simulink model "plane"  (R2023b)
settings: Solver=FixedStepDiscrete  StartTime=0.0  StopTime=17.0  FixedStep=1  RelTol=1e-3  EnableMultiTasking=on
libraries: simulink x3
settings Model: Creator=yueyue  LastModifiedBy=yueyue

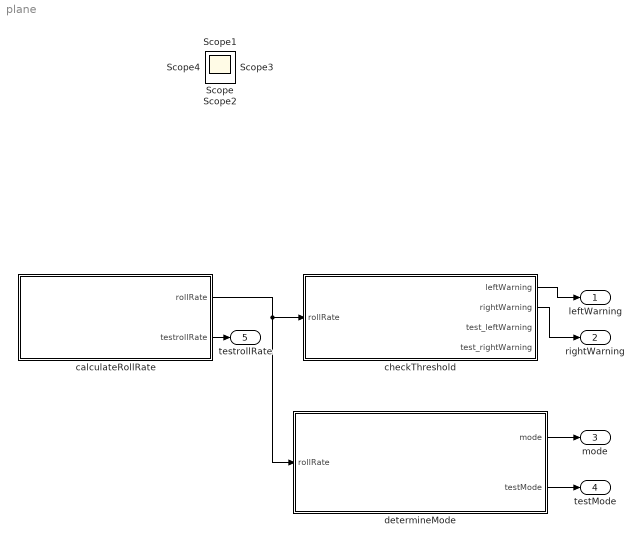
== system plane ==
  calculateRollRate : Subsystem
  checkThreshold : Subsystem
  determineMode : Subsystem
  leftWarning : Outport
  rightWarning : Outport  Port=2
  mode : Outport  Port=3
  testMode : Outport  Port=4
  testrollRate : Outport  Port=5
  Scope{,1..4} (5 alike) : Scope
  wires:
  calculateRollRate/1(rollRate) -> determineMode/1(rollRate), checkThreshold/1(rollRate)
  checkThreshold/1(leftWarning) -> leftWarning/1
  checkThreshold/2(rightWarning) -> rightWarning/1
  determineMode/1(mode) -> mode/1
  determineMode/2(testMode) -> testMode/1
  calculateRollRate/2(testrollRate) -> testrollRate/1

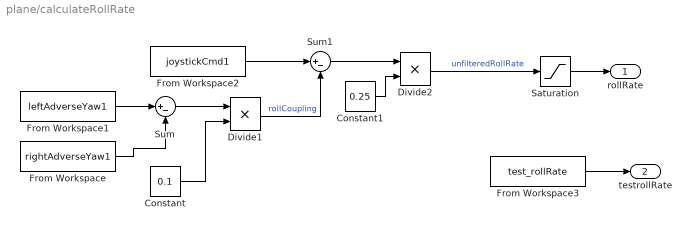
== system plane/calculateRollRate ==
  Constant : Constant  Value=0.1
  Constant1 : Constant  Value=0.25
  Divide1 : Product  Inputs=**
  Divide2 : Product  Inputs=**
  From Workspace : FromWorkspace  VariableName=rightAdverseYaw1  SampleTime=1
  From Workspace1 : FromWorkspace  VariableName=leftAdverseYaw1  SampleTime=1
  From Workspace2 : FromWorkspace  VariableName=joystickCmd1  SampleTime=1
  From Workspace3 : FromWorkspace  VariableName=test_rollRate  SampleTime=1
  Saturation : Saturate  UpperLimit=25.0  LowerLimit=-25.0  ZeroCross=off
  Sum : Sum  Inputs=|+-
  Sum1 : Sum  Inputs=|+-
  rollRate : Outport
  testrollRate : Outport  Port=2
  wires:
  Sum/1 -> Divide1/1
  Constant/1 -> Divide1/2
  Divide1/1 -> Sum1/2  "rollCoupling"
  Sum1/1 -> Divide2/1
  Constant1/1 -> Divide2/2
  Divide2/1 -> Saturation/1  "unfilteredRollRate"
  Saturation/1 -> rollRate/1
  From Workspace/1 -> Sum/2
  From Workspace1/1 -> Sum/1
  From Workspace2/1 -> Sum1/1
  From Workspace3/1 -> testrollRate/1

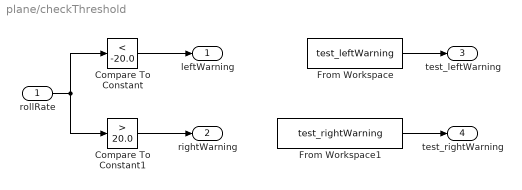
== system plane/checkThreshold ==
  rollRate : Inport
  Compare To Constant : simulink/Logic and Bit Operations/Compare To Constant  relop=<  const=-20.0  OutDataTypeStr=boolean
  Compare To Constant1 : simulink/Logic and Bit Operations/Compare To Constant  relop=>  const=20.0  OutDataTypeStr=boolean
  From Workspace : FromWorkspace  VariableName=test_leftWarning  SampleTime=1
  From Workspace1 : FromWorkspace  VariableName=test_rightWarning  SampleTime=1
  leftWarning : Outport
  rightWarning : Outport  Port=2
  test_leftWarning : Outport  Port=3
  test_rightWarning : Outport  Port=4
  wires:
  rollRate/1 -> Compare To Constant/1, Compare To Constant1/1
  Compare To Constant/1 -> leftWarning/1
  Compare To Constant1/1 -> rightWarning/1
  From Workspace/1 -> test_leftWarning/1
  From Workspace1/1 -> test_rightWarning/1

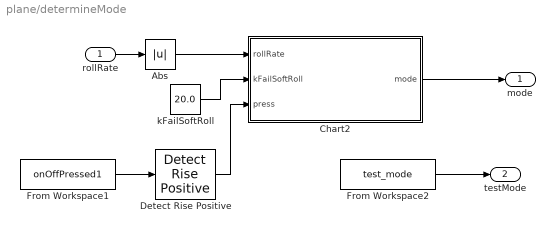
== system plane/determineMode ==
  rollRate : Inport
  Abs : Abs  SaturateOnIntegerOverflow=off
  Chart2 : Stateflow chart  TreatAsAtomicUnit=on
  Detect Rise Positive : simulink/Logic and Bit Operations/Detect Rise Positive  vinit=1  OutDataTypeStr=boolean
  From Workspace1 : FromWorkspace  VariableName=onOffPressed1  SampleTime=1
  From Workspace2 : FromWorkspace  VariableName=test_mode  SampleTime=1
  kFailSoftRoll : Constant  Value=20.0
  mode : Outport
  testMode : Outport  Port=2
  wires:
  From Workspace1/1 -> Detect Rise Positive/1
  Chart2/1(mode) -> mode/1
  Abs/1 -> Chart2/1(rollRate)
  rollRate/1 -> Abs/1
  kFailSoftRoll/1 -> Chart2/2(kFailSoftRoll)
  Detect Rise Positive/1 -> Chart2/3(press)
  From Workspace2/1 -> testMode/1

== stateflow chart plane/determineMode/Chart2 ==
  settings: executeAtInitialization=1
  state Off
    entry:
    mode=0;
  state ON
    state FailSoft
      entry:
      mode=2;
    state Nominal
      entry:
      mode=1;
    (default) -> (junction 43)
    (junction 43) -> FailSoft [order 2]
    (junction 43) -> Nominal [order 1] : [rollRate<=kFailSoftRoll]
    Nominal -> FailSoft : [rollRate>kFailSoftRoll]
    FailSoft -> Nominal : [rollRate<=kFailSoftRoll]
  (default) -> Off
  Off -> ON : [press]
  ON -> Off : [press]
  data: rollRate input; kFailSoftRoll input; mode output; press input
